simulink library "RxFloatingPointLibrary"  (R2019b)
settings: Solver=VariableStepAuto  StartTime=0.0  StopTime=10.0  RelTol=1e-3
undefined symbols (not defined in the file): crcDecodeLag, magnitude, numTrainingSamples, RadioSampleRate, samplesPerSymbol, VibertiTracebackLength, xPreambleSeq
libraries: simulink x16, hdlsllib x2, commdigbbndpm3 x2, commcrc2 x1, dspstat3 x1, dspsigops x1, commseqgen3 x1, commcnvcod2 x1, commutil2 x1, commfilt2 x1
(part 2 of 2)

== matlab function RxFloatingPointLibrary/Receiver/CRC Check and DMA Pack/CRC Check ES/Debug CRC input ==
  data: u input; enable input; endFlag input; startFlag input
function fcn(u, enable,endFlag,startFlag)

persistent buffer crc count

if isempty(buffer)
   buffer = false(1700,1); 
    crc = comm.CRCDetector('Polynomial','z^32 + z^26 + z^23 + z^22 + z^16 + z^12 + z^11 + z^10 + z^8 + z^7 + z^5 + z^4 + z^2 + z + 1');
    count = 1;
end

if enable
    %buffer = [buffer(2:end);u];
    if startFlag
        count = 1;
    elseif count>1700-1
        count = 1;
    else
        count = count + 1;
    end
    buffer(count) = u;
    
    if endFlag
        disp(count)
        k = buffer(1:1632);
        [~,e] = crc(k);
        if e
            disp('Error');
        else
            disp('Pass');
        end
    end
    
end

== matlab function RxFloatingPointLibrary/Receiver/Frame Recover/Enable Equalizer and Packet Decode (Latch) ==
  data: start input; enable output; validIn input
function enable = Counter(start,validIn)

persistent count maxCount lastEOF

if isempty(count)
    count = 0;
    maxCount = 2^16; % Largest possible packet length
    lastEOF = false;
end

eof = false;

if validIn
    % Got a barker preamble start allowing data into equalizer
    if start
        count = maxCount;
    end
    
    % Check on change from true to false
    if lastEOF && ~eof
        %     fprintf('Frame end reached\n');
        count = 0;
    end
    lastEOF = eof;
    
    % Past end of max frame size
    if count>0
        count = count - 1;
    end
    
    % Enable downstream
    enable = count>0;
else
    enable = false;
end

== matlab function RxFloatingPointLibrary/Receiver/Frame Recover/Equalization and Demodulation/Descrambler1/MATLAB Function ==
  data: data input; vec output; reset input
function vec = ResetableTapDelay(data,reset)

persistent buffer

if isempty(buffer)
    buffer = [0 1 0 0 0 1 0]>0;
end
    
if reset
    vec = [0 1 0 0 0 1 0]>0;
    buffer = [0 1 0 0 0 1 0]>0;
else
   vec = [buffer(2:end),data];
   buffer = [buffer(2:end),data];
end

== matlab function RxFloatingPointLibrary/Receiver/CRC Check and DMA Pack/CRC Check ES/Check CRC Result (DEBUG) ==
  data: bits input; start input; done input; valid input; err input
function fcn(bits, start, done, valid, err)

persistent buffer

if isempty(buffer)
    buffer = fi(false(1032,1),0,1,0);
end

buffer = [buffer(2:end);bits];

if done && valid
    if err
        fprintf('CRC Error (HDL CRC)\n');
    else
        fprintf('CRC Passed (HDL CRC)\n');
    end
end
if err % Flag if any error every occurs, if it occurs alone it means given crc is not long enough
    fprintf('CRC Error Type 2 (HDL CRC)\n');
end

== matlab function RxFloatingPointLibrary/Receiver/Frame Recover/Equalization and Demodulation/DFE/Equalizer ==
  data: trigger input; eqOut output; data input; trainingSymbol input; ec output
function [eqOut,ec]  = dfe(trigger,data,trainingSymbol)

persistent inputBuffer decisionBuffer forwardTaps backwardTaps processedSamples


%% Constants
WL = uint8(16); FL = uint8(14);
F = fimath('SumMode','SpecifyPrecision','SumWordLength',WL,...
    'SumFractionLength',FL);
% Initial delay guess
channelDelay = uint8(0);
% Equalizer settings
mu = fi(0.05,0,10,12);
nFTaps = uint8(11);
nBTaps = uint8(3);
numTrainingSymbols = uint16(250);
resetTaps = fi([complex(zeros(nFTaps-1,1));1],1,WL,FL,F);

%% Async
if isempty(inputBuffer)
    % Set Precisions
    inputBuffer = fi(complex(zeros(nFTaps,1)),1,WL,FL,F);
    decisionBuffer = fi(complex(zeros(nBTaps,1)),1,WL,FL,F);
    forwardTaps = fi(complex(zeros(nFTaps,1)),1,WL,FL,F);
    backwardTaps = fi(complex(zeros(nBTaps,1)),1,WL,FL,F);
    processedSamples = numTrainingSymbols + uint16(1); % Force to DD mode to start
end

%% Reset
if trigger
    processedSamples = uint16(0);
    % Reset taps
    %forwardTaps = fi(complex(zeros(nFTaps,1)),1,WL,FL,F);
    %forwardTaps(nFTaps-channelDelay) = fi(1,1,WL,FL); % Favor specific delay (causes equalizer to converge faster)
    forwardTaps = resetTaps;
    backwardTaps = fi(complex(zeros(nBTaps,1)),1,WL,FL,F);
    % Default output
    eqOut = fi(complex(0),1,WL,FL,F);
    ec = fi(complex(0),1,WL,FL,F);
else
    %% Equalizer
    % Add data to buffer
    inputBuffer = [inputBuffer(2:end);data];
    
    % Apply equalizer
    eqOut = forwardTaps'*inputBuffer - backwardTaps'*decisionBuffer;
    
    % Determine error
    if (processedSamples<numTrainingSymbols) && (processedSamples>=channelDelay)
        processedSamples = processedSamples + 1;
        d = trainingSymbol;
    else % Decision directed
        % Find closest symbol
        r = real(eqOut)>0; i = imag(eqOut)>0;
        if r
            if i
                d = fi(0.7071 + 0.7071i,1,WL,FL);
            else
                d = fi(0.7071 - 0.7071i,1,WL,FL);
            end
        else
            if i
                d = fi(-0.7071 + 0.7071i,1,WL,FL);
            else
                d = fi(-0.7071 - 0.7071i,1,WL,FL);
            end
        end
    end
    ec = conj(d - eqOut);
    
    % Update taps
    forwardTaps = forwardTaps + mu*ec*inputBuffer;
    backwardTaps = backwardTaps - mu*ec*decisionBuffer;
    
    % Update decision buffer
    db = fi(d,1,WL,FL,F);
    decisionBuffer = [db; decisionBuffer(1:end-1)];
    
end



end

== matlab function RxFloatingPointLibrary/Receiver/Frame Recover/Frequency Recovery/PED ==
  data: In input; e output
function e  = PED(In)


e = sign(real(In)).*imag(In) - sign(imag(In)).*real(In);

== matlab function RxFloatingPointLibrary/Receiver/Frame Recover/Barker Locate/Measure Phase Ambiguity/Get Index of max ==
  data: noShift input; shift output; pi4 input; pi2 input; pi34 input; trigger input
function shift = DetermineShift(noShift, pi4, pi2, pi34, trigger)
%#codegen

persistent rotation available

if isempty(rotation)
    rotation = 1;
    available = exp(-(0:pi/2:(pi*3/2)) .* 1i);
end

if trigger
[~,i] = max(imag([noShift, pi4, pi2, pi34]));
rotation = available(i);
end


shift = rotation;

== matlab function RxFloatingPointLibrary/Receiver/CRC Check and DMA Pack/DMA Interface/Bit Packer ==
  data: bitIn input; byteOut output; startIn input; endIn input; err input; validIn input; validOut output; startOut output
function [byteOut,validOut,startOut] = BitPacker(bitIn, startIn, endIn, err, validIn)

% This block will pack bits into bytes with start boundaries


% Constants
bits2Pack = uint8(64); % byteReg must contain this many bits
% NOTE: Frames but be a multiple of bits2Pack or bits will be trimmed from
% end

persistent byteReg byteIndx setStartFlag

if isempty(byteIndx)
    byteReg  = fi(0,0,64,0);
    byteIndx = uint8(1);
    setStartFlag = false;
end

if validIn
    if startIn % Reset
        bitset(byteReg,1,bitIn);
        byteIndx = uint8(2);
        validOut = false;
        setStartFlag = true;
        startOut = false;
    else
        byteReg = bitset(byteReg,byteIndx,bitIn);
        if byteIndx >= bits2Pack
            byteIndx = uint8(1);
            validOut = true;
            startOut = setStartFlag;
            setStartFlag = false;
        else
            byteIndx = byteIndx + uint8(1);
            validOut = false;
            startOut = false;
        end
    end
elseif endIn % Append error bit to last byte
    byteReg = fi(err,0,64,0);
    validOut = true;
    startOut = false;
else
    validOut = false;
    startOut = false;
end

byteOut = byteReg;

== matlab function RxFloatingPointLibrary/Receiver/CRC Check and DMA Pack/overdrive ==
  data: validIn input; enableCRC output; endIn input
function enableCRC = fcn(validIn,endIn)

% This block drives the enabled subsystem an additional step so the
% outputs do not stay high but reset.  All signals are reset since the
% driving valid signal is false

persistent gotEndOut

if isempty(gotEndOut)
    gotEndOut = false;
end
    
if validIn
    enableCRC = true;
    gotEndOut = false;
else
    if endIn
        gotEndOut = true;
        enableCRC = true;
    elseif gotEndOut
        enableCRC = true;
    else
        enableCRC = false;
    end
end

== matlab function RxFloatingPointLibrary/Receiver/Frame Recover/Equalization and Demodulation/Find packet tail and check CRC (DEBUG ONLY AND REQUIRES TAIL BITS) ==
  data: u input
function findTail(u)

persistent tailBits buffer counter head

if isempty(tailBits)
   tailBits = repmat(uint8([1 0 1 1 0 0 1 1 1 1].'),4,1);
   buffer = uint8(zeros(size(tailBits)));
    counter = 0;
    head = uint8(ones(16,1));
end

%buffer = [u; buffer(1:end-1)];
buffer = [buffer(2:end); u];
counter = counter + 2; % Coded bit counter

% Check for tail sequence
found = 0;
if isequal(buffer,tailBits)
   fprintf('Found tail after %d coded bits\n',int64(counter));
   counter = 0;
   found = 1;
end

%% CHECK CRC
persistent crc buffer2
CRCLen = 32;
nPayLoad = 8*200;
nTB = length(tailBits);

if isempty(crc)
    crc = comm.CRCDetector('Polynomial','z^32 + z^26 + z^23 + z^22 + z^16 + z^12 + z^11 + z^10 + z^8 + z^7 + z^5 + z^4 + z^2 + z + 1');
    buffer2 = false(CRCLen+nPayLoad+nTB,1);%false(10532+40,1);
end

crcCase = 0;
enable = false;

buffer2 = [buffer2(2:end); u>0];
%if isequal(head, buffer2(end-15:end))
%   fprintf('Head FOUND %d\n',int64(counter));
%end
if found>0
    NoTailBits = buffer2(1:end-nTB);
    PayloadWithCRC= NoTailBits(end-nPayLoad-CRCLen+1:end);
    enable = true;
    [~,e] = crc(PayloadWithCRC);
    if ~e
        crcCase = 1;
        fprintf('Packet CRC Passed\n');
    else
        crcCase = 0;
        fprintf('Packet CRC Failed\n');
    end
    
end

== matlab function RxFloatingPointLibrary/Receiver/Frame Recover/Equalization and Demodulation/Header Controller ==
  data: headerStart input; enableDownstream output; packetLenBitsOut output; data input; resetViterbi output; crcStart output
function [enableDownstream,packetLenBitsOut,resetViterbi,crcStart] = EvalHeader(headerStart, data)

persistent counter sum1 sum2 packetLenBits lastMode savedPacketLenBits

% The header contains 16 bits, but each bit is duplicated to make checking
% easier

% Note this block works on symbols (2bits) but 1 symbol -> 1 decoded bit

% PacketLength = (Data+CRC+40(TB)+68)/CodeRate

% NOTE TAIL BITS HERE ARE REALLY USED TO DEAL WITH VITERBI LAG SO:
% TailBitsWithLagPadding > TracebackLength

%% Constants
numHeaderBits = 16; % Header is this many bits
%TracebackLength = 34+20;
%CRCLen = 32;
CodeRateINV = 2;%1/CodeRate;
TailBitsWithLagPadding = 40+34*2+1;
% Flag when CRC porition of packet starts relative to header
%crcSignalStartLocation = uint32((TailBitsWithLagPadding+CRCLen)*CodeRateINV); % Must be even
crcSignalStartLocation = (TailBitsWithLagPadding)*CodeRateINV; % Must be even

%% Async/Initialization
if isempty(counter)
    packetLenBits = 0;
    sum1 = uint32(0);
    sum2 = uint32(0);
    counter = numHeaderBits;
    lastMode = 3;
    savedPacketLenBits = 0;
end

%% Sync
switch lastMode
    %% Reset on preamble flag and setup for header processing
    case 0
        crcStart = false;
        resetViterbi = false;
        enableDownstream = false;
        sum1 = uint32(0);
        sum2 = uint32(0);
        counter = 1;
        lastMode = 1; % Go to next state
        packetLenBitsOut = 0;
        
    %% Process header
    case 1 
        crcStart = false;
        enableDownstream = false;
        
        % Convert header bits (bit by bit)
        sum1 = bitset(sum1,counter,data(1));
        sum2 = bitset(sum2,counter,~data(2));
        counter = counter + 1;
        
        if counter>numHeaderBits
            % Check header
            if sum1~=sum2 % Fail
                packetLenBits = 0;
                lastMode = 3;
                resetViterbi = false;
                packetLenBitsOut = 0;
                savedPacketLenBits = 0;
                fprintf('Header Check failed (possible false detection)\n');
                fprintf('sum1: %d\n',int32(sum1));
                fprintf('sum2: %d\n',int32(sum2));
            else % Pass
                % Saved header info and trigger downstream
                packetLenBits = double(sum1);
                lastMode = 2;
                resetViterbi = true;
                packetLenBitsOut = (double(sum1)-crcSignalStartLocation);
                savedPacketLenBits = (double(sum1)-crcSignalStartLocation);
                fprintf('Header Found | Packet is %d bits long\n',int32(sum1));            
            end
        else
            packetLenBitsOut = 0;
            resetViterbi = false;
        end
        
    %% Decrement sample counter
    case 2 
        resetViterbi = false;
        crcStart = (packetLenBits==crcSignalStartLocation);
        if packetLenBits>uint32(0)
            enableDownstream = true;
            packetLenBits = packetLenBits - 2; % We get 2 bits each call
            packetLenBitsOut = savedPacketLenBits;
        else
            enableDownstream = false;
            savedPacketLenBits = 0;%Reset
            packetLenBitsOut = 0; %Reset
            lastMode = 3;
        end
            
    %% Not processing anything
    otherwise % mode>2
        crcStart = false;
        resetViterbi = false;
        enableDownstream = false;
        packetLenBitsOut = 0;
end

%% Got a header now reset to mode 0 on next call
if headerStart
    lastMode = 0; % Go to reset mode
end

%%

% % Set default flags, which may change
% resetViterbi = false;
% crcStart = false;
% 
% % Reset when preamble found (barker sequence)
% if headerStart
%     sum1 = uint32(0);
%     sum2 = uint32(0);
%     counter = uint32(1);
% end
% 
% % Send data downstream to
% enableDownstream = packetLenBits>uint32(0);
% 
% % Flag when we are in CRC section of packet
% % Enable signal will relate to first bit of CRC portion of packet
% if packetLenBits==crcSignalStartLocation
%     crcStart = true;
% end
% 
% % Decrement packet length counter
% if enableDownstream
%     packetLenBits = packetLenBits - uint32(2); % Get 2 bits each call
% end
% 
% % Process header
% if counter<=headerBits
%     % Convert header bits (bit by bit)
%     if data(1)
%         sum1 = sum1 + powersOfTwo(counter);
%     end
%     if data(2)
%         sum2 = sum2 + powersOfTwo(counter);
%     end
%     counter = counter + uint32(1);
%     
%     if counter>headerBits
%         % Check header
%         if sum1~=sum2
%             packetLenBits = uint32(0);
%             enableDownstream = false;
%             fprintf('Header Check failed (possible false detection)\n');
%         else
%             % Saved header info and trigger downstream
%             packetLenBits = uint32(sum1);
%             fprintf('Header Found | Packet is %d bits long\n',int32(sum1));
%             resetViterbi = true;
%             enableDownstream = true;
%         end
%     end
%     
% end
